simulink model "MCC_boucle_ouverte"  (R2024a)
settings: Solver=ode45  StartTime=0.0  StopTime=Tfinal  RelTol=1e-3
undefined symbols (not defined in the file): A, B_sim, C, D_sim, Tmec, Va, x0
settings Model: Creator=DELL  LastModifiedBy=DELL

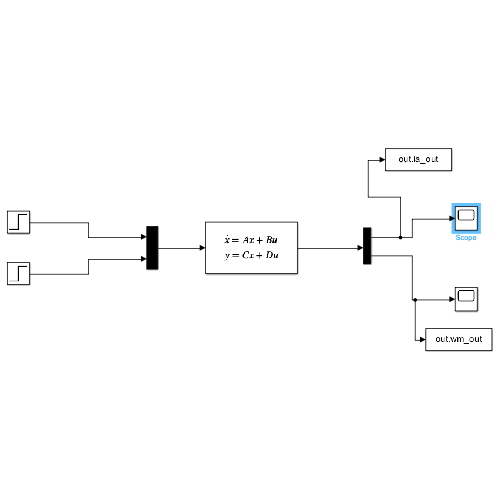
[thumbnail: Simulink's stored preview of the top-level diagram]
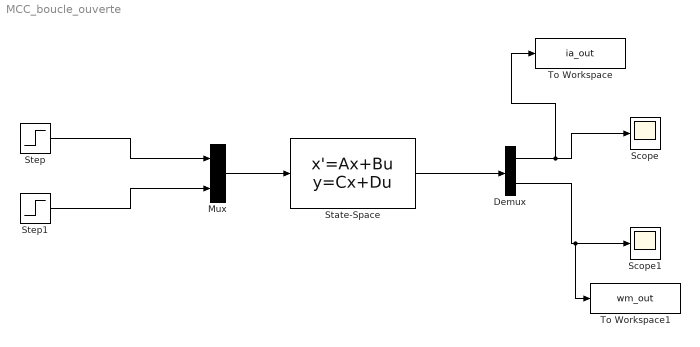
== system MCC_boucle_ouverte ==
  Demux : Demux  Outputs=2
  Mux : Mux  Inputs=2
  Scope : Scope
  Scope1 : Scope
  State-Space : StateSpace  A=A  B=B_sim  C=C  D=D_sim  InitialCondition=x0
  Step : Step  Time=0.1  After=Va  SampleTime=0
  Step1 : Step  Time=0.5  After=Tmec  SampleTime=0
  To Workspace : ToWorkspace  VariableName=ia_out  SaveFormat=Timeseries  SampleTime=-1
  To Workspace1 : ToWorkspace  VariableName=wm_out  SaveFormat=Timeseries  SampleTime=-1
  wires:
  Mux/1 -> State-Space/1
  State-Space/1 -> Demux/1
  Step/1 -> Mux/1
  Step1/1 -> Mux/2
  Demux/1 -> To Workspace/1, Scope/1
  Demux/2 -> To Workspace1/1, Scope1/1
